simulink library "INT_CEngDsT_VD"  (R2016b)
settings: Solver=VariableStepAuto  StartTime=0.0  StopTime=10.0  RelTol=1e-3
settings Model: Creator=dulinggang  LastModifiedBy=dulinggang

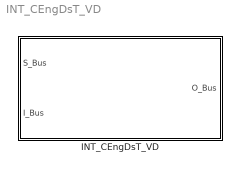
== system INT_CEngDsT_VD ==
  INT_CEngDsT_VD : Subsystem

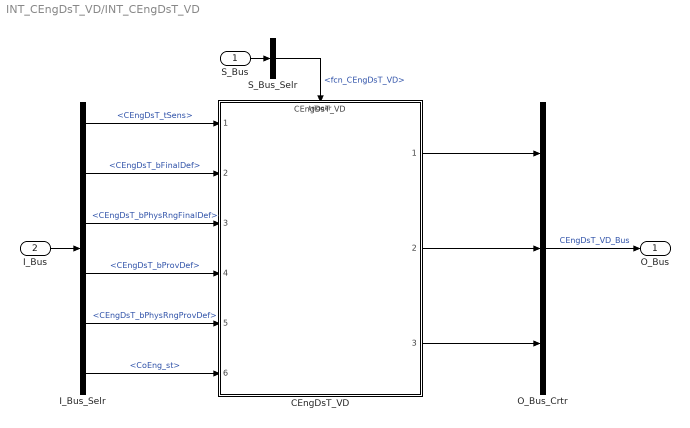
== system INT_CEngDsT_VD/INT_CEngDsT_VD ==
  S_Bus : Inport
  I_Bus : Inport  Port=2
  CEngDsT_VD : ModelReference  ModelNameDialog=CEngDsT_VD  SimulationMode=Normal  ModelReferenceVersion=1.126  TriggerPortName=function  TriggerPortTriggerType=function-call  TriggerPortStatesWhenEnabling=held
  I_Bus_Selr : BusSelector  OutputSignals=CEngDsT_tSens,CEngDsT_bFinalDef,CEngDsT_bPhysRngFinalDef,CEngDsT_bProvDef,CEngDsT_bPhysRngProvDef,CoEng_st
  O_Bus_Crtr : BusCreator  Inputs=3
  S_Bus_Selr : BusSelector  OutputSignals=fcn_CEngDsT_VD
  O_Bus : Outport
  wires:
  S_Bus_Selr/1 -> CEngDsT_VD/Trigger  "<fcn_CEngDsT_VD>"
  S_Bus/1 -> S_Bus_Selr/1
  I_Bus/1 -> I_Bus_Selr/1
  I_Bus_Selr/1 -> CEngDsT_VD/1  "<CEngDsT_tSens>"
  I_Bus_Selr/2 -> CEngDsT_VD/2  "<CEngDsT_bFinalDef>"
  I_Bus_Selr/3 -> CEngDsT_VD/3  "<CEngDsT_bPhysRngFinalDef>"
  I_Bus_Selr/4 -> CEngDsT_VD/4  "<CEngDsT_bProvDef>"
  I_Bus_Selr/5 -> CEngDsT_VD/5  "<CEngDsT_bPhysRngProvDef>"
  I_Bus_Selr/6 -> CEngDsT_VD/6  "<CoEng_st>"
  O_Bus_Crtr/1 -> O_Bus/1  "CEngDsT_VD_Bus"
  CEngDsT_VD/1 -> O_Bus_Crtr/1
  CEngDsT_VD/2 -> O_Bus_Crtr/2
  CEngDsT_VD/3 -> O_Bus_Crtr/3
